simulink model "Ass5_extra"  (R2024b)
settings: Solver=FixedStepAuto  StartTime=0.0  StopTime=inf  FixedStep=dt  RelTol=1e-3
model workspace (MATLAB code in the model file):
  | dt=0.2;
libraries: simulink x1
settings Model: SnapshotBufferSize=100  SnapshotInterval=100  PacingRate=5  Creator=ArriGE66  LastModifiedBy=vise
settings ModelReferenceCC: EnableRefExpFcnMdlSchedulingChecks=on
settings RTWCC: GPUComputeCapability=3.5

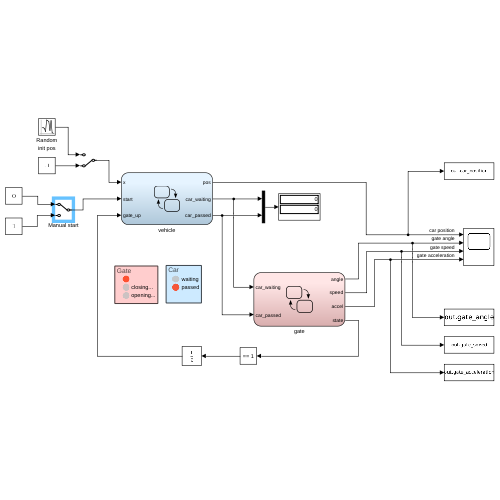
[thumbnail: Simulink's stored preview of the top-level diagram]
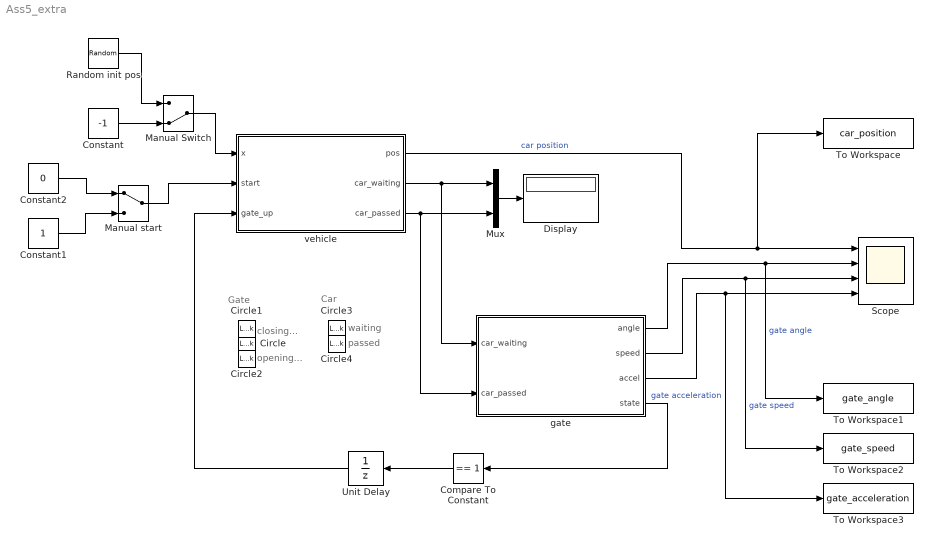
== system Ass5_extra ==
  note: Car
  note: waiting
  note: Gate
  note: closing...
  note: opening...
  note: passed
  Circle{,1..4} (5 alike) : LampBlock  LabelPosition=Hide  Icon=Circle
  Compare To Constant : simulink/Logic and Bit Operations/Compare To Constant  relop===  const=1  OutDataTypeStr=boolean
  Constant : Constant  Value=-1
  Constant1 : Constant
  Constant2 : Constant  Value=0
  Display : Display
  Manual Switch : ManualSwitch  CurrentSetting=0
  Manual start : ManualSwitch
  Mux : Mux  Inputs=2
  Random init pos : RandomNumber  Mean=-15  Variance=5
  Scope : Scope  NumInputPorts=4
  To Workspace : ToWorkspace  VariableName=car_position  SampleTime=-1
      settings: Save2DSignal=2-D array (concatenate along first dimension)
  To Workspace1 : ToWorkspace  VariableName=gate_angle  SampleTime=-1
      settings: Save2DSignal=2-D array (concatenate along first dimension)
  To Workspace2 : ToWorkspace  VariableName=gate_speed  SampleTime=-1
      settings: Save2DSignal=2-D array (concatenate along first dimension)
  To Workspace3 : ToWorkspace  VariableName=gate_acceleration  SampleTime=-1
      settings: Save2DSignal=2-D array (concatenate along first dimension)
  Unit Delay : UnitDelay  SampleTime=-1  HasFrameUpgradeWarning=on
  gate : Stateflow chart  TreatAsAtomicUnit=on
  vehicle : Stateflow chart  TreatAsAtomicUnit=on
  wires:
  Constant1/1 -> Manual start/2
  Constant2/1 -> Manual start/1
  Manual start/1 -> vehicle/2(start)
  Compare To Constant/1 -> Unit Delay/1
  vehicle/1(pos) -> To Workspace/1, Scope/1  "car position"
  Mux/1 -> Display/1
  vehicle/3(car_passed) -> gate/2(car_passed), Mux/2
  vehicle/2(car_waiting) -> gate/1(car_waiting), Mux/1
  gate/4(state) -> Compare To Constant/1
  Unit Delay/1 -> vehicle/3(gate_up)
  Random init pos/1 -> Manual Switch/1
  Manual Switch/1 -> vehicle/1(x)
  Constant/1 -> Manual Switch/2
  gate/3(accel) -> To Workspace3/1, Scope/4  "gate acceleration"
  gate/2(speed) -> To Workspace2/1, Scope/3  "gate speed"
  gate/1(angle) -> Scope/2, To Workspace1/1  "gate angle"

== stateflow chart Ass5_extra/gate ==
  state Closed
    angle=0;
    speed=0;
    accel=0;
    state=0;
  state Opening
    state=2;
    state phaseB
      t=elapsed(sec)+dt;
      accel=0;
      speed=4;
      angle=8+speed*t;
    state phaseA
      t=elapsed(sec)+dt;
      accel=1;
      speed=accel*t;
      angle=0.5*accel*t^2
    state phaseC
      t=elapsed(sec)+dt;
      accel=-1;
      speed=4+accel*t;
      angle=4*t+82+0.5*accel*t^2
    (default) -> Opening.phaseA
    Opening.phaseA -> Opening.phaseB : [angle>=8]
    Opening.phaseB -> Opening.phaseC : [angle>=82]
  state CaseC
    state=2;
    state phaseB
      t=elapsed(sec)+dt;
      accel=0;
      speed=4;
      angle=in_angle+speed*t;
    state phaseA
      t=elapsed(sec)+dt;
      accel=1;
      speed=in_speed+accel*t;
      angle=in_angle+in_speed*t+0.5*accel*t^2
    state phaseC
      t=elapsed(sec)+dt;
      accel=-1;
      speed=4+accel*t;
      angle=4*t+82+0.5*accel*t^2
    (default) -> CaseC.phaseA
    CaseC.phaseA -> CaseC.phaseB : [speed>=4]
    CaseC.phaseB -> CaseC.phaseC : [angle>=82]
  state Closing
    state=3;
    state phaseB
      t=elapsed(sec)+dt;
      accel=0;
      speed=-4;
      angle=82+speed*t;
    state phaseA
      t=elapsed(sec)+dt;
      accel=-1;
      speed=accel*t;
      angle=90+0.5*accel*t^2
    state phaseC
      t=elapsed(sec)+dt;
      accel=1;
      speed=-4+accel*t;
      angle=-4*t+8+0.5*accel*t^2
    (default) -> Closing.phaseA
    Closing.phaseA -> Closing.phaseB : [angle<=82]
    Closing.phaseB -> Closing.phaseC : [angle<=8]
  state Open
    angle=90;
    speed=0;
    accel=0;
    state=1;
  (default) -> Closed
  Closing -> Closed [order 1] : [speed==0 && angle<=8]
  Closed -> Opening : [car_waiting==1]
  Closing -> CaseC [order 2] : [car_waiting==1 && angle<=82]
      | {in_speed=speed; in_angle=angle}
  Open -> Closing : [car_passed==1]
  CaseC -> Open : [speed==0 && angle>=82]
  Opening -> Open : [speed==0 && angle>=82]
  data: car_waiting input; angle output; speed output; accel output; state output; t local; dt parameter double; car_passed input; in_angle local; in_speed local

== stateflow chart Ass5_extra/vehicle ==
  state idle
    init=x;
    pos=init;
    car_waiting=0;
    car_passed=0;
  state approaching
    pos=init+v*elapsed(sec);
  state stop
    tmp=pos;
    car_waiting=1;
    car_passed=0;
  state pass
    pos=tmp+v*elapsed(sec);
    car_waiting=0;
    ex:
    pos=tmp+v*elapsed(sec);
    tmp=pos;
  state passed
    pos=tmp+v*elapsed(sec);
    car_passed=1;
  (default) -> idle
  approaching -> stop : [pos>=0]
  idle -> approaching : [start==1]
  passed -> idle : [after(1,sec)]
  stop -> pass : [gate_up==1]
  pass -> passed : [pos>= gate_end]
  data: gate_end local =3; v local double =1; pos output; car_waiting output; car_passed output; init local; x input; start input; gate_up input; tmp local
